simulink model "LAB_2"  (R2021a)
settings: Solver=VariableStepAuto  StartTime=0.0  StopTime=10.0  RelTol=1e-3
settings Model: Creator=hp  LastModifiedBy=hp

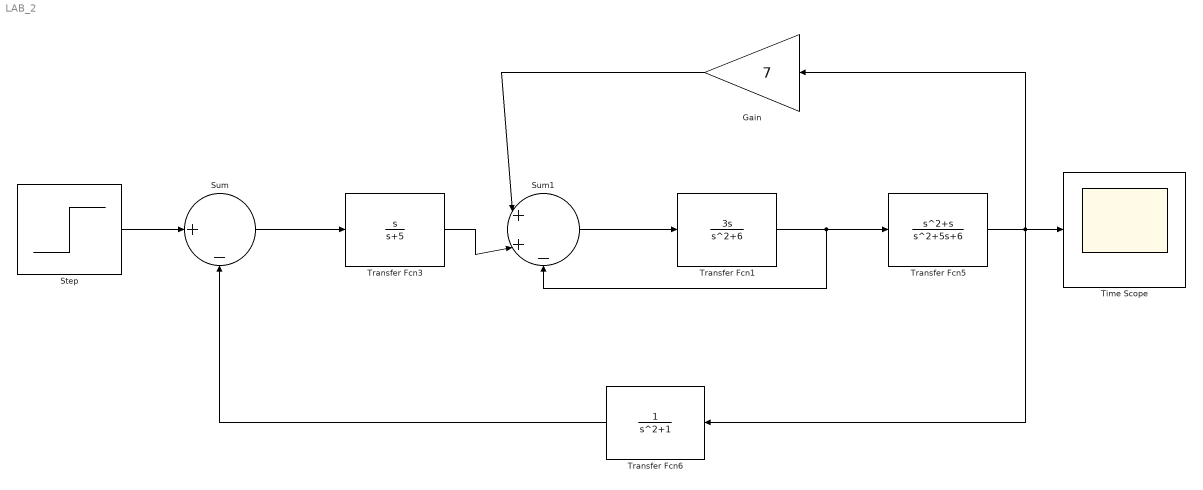
== system LAB_2 ==
  Gain : Gain  Gain=7
  Step : Step  SampleTime=0
  Sum : Sum  Inputs=|+-
  Sum1 : Sum  Inputs=|++-
  Time Scope : Scope
  Transfer Fcn1 : TransferFcn  Numerator=[3 0]  Denominator=[1 0 6]
  Transfer Fcn3 : TransferFcn  Numerator=[1 0]  Denominator=[1 5]
  Transfer Fcn5 : TransferFcn  Numerator=[1 1 0]  Denominator=[1 5 6]
  Transfer Fcn6 : TransferFcn  Denominator=[1 0 1]
  wires:
  Step/1 -> Sum/1
  Sum/1 -> Transfer Fcn3/1
  Sum1/1 -> Transfer Fcn1/1
  Transfer Fcn1/1 -> Sum1/3, Transfer Fcn5/1
  Transfer Fcn5/1 -> Transfer Fcn6/1, Gain/1, Time Scope/1
  Transfer Fcn3/1 -> Sum1/2
  Gain/1 -> Sum1/1
  Transfer Fcn6/1 -> Sum/2
